simulink library "uavsimBlockset_UAV3D_visualizeBox"  (Simulink 8.6)
settings: Solver=ode45  StartTime=0.0  StopTime=10.0  RelTol=1e-3
libraries: aerolibtransform2 x1, uavsimBlockset_UAV3DInterface x1
settings Model: Creator=mstolle  LastModifiedBy=j.bolting

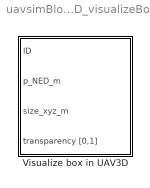
== system uavsimBlockset_UAV3D_visualizeBox ==
  Visualize box in UAV3D : Subsystem  TreatAsAtomicUnit=on  SystemSampleTime=1/10

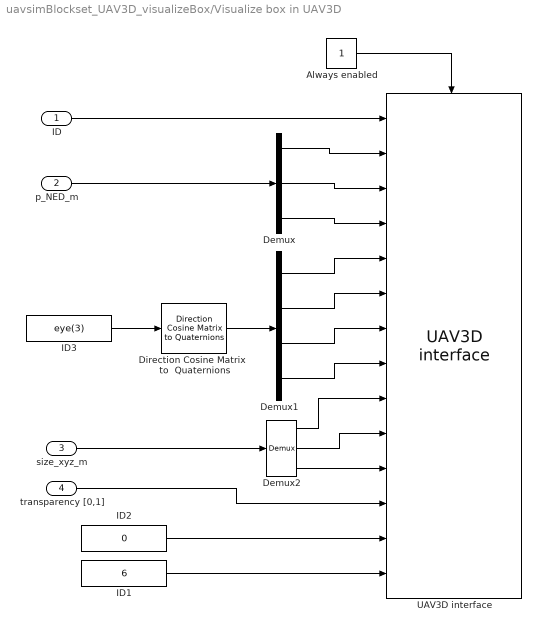
== system uavsimBlockset_UAV3D_visualizeBox/Visualize box in UAV3D ==
  ID : Inport
  p_NED_m : Inport  Port=2
  size_xyz_m : Inport  Port=3
  transparency [0,1] : Inport  Port=4
  Always enabled : Constant
  Demux : Demux  Outputs=3
  Demux1 : Demux
  Demux2 : Demux  Outputs=3
  Direction Cosine Matrix   to  Quaternions : aerolibtransform2/Direction Cosine Matrix  to Quaternions
  ID1 : Constant  Value=6
  ID2 : Constant  Value=0
  ID3 : Constant  Value=eye(3)
  UAV3D interface : uavsimBlockset_UAV3DInterface/UAV3D interface  ip='localhost'  udpport=4445
  wires:
  Always enabled/1 -> UAV3D interface/Enable
  transparency [0,1]/1 -> UAV3D interface/12
  Demux1/1 -> UAV3D interface/5
  Demux/2 -> UAV3D interface/3
  Demux/1 -> UAV3D interface/2
  Demux/3 -> UAV3D interface/4
  Demux1/2 -> UAV3D interface/6
  Demux1/3 -> UAV3D interface/7
  Demux1/4 -> UAV3D interface/8
  ID1/1 -> UAV3D interface/14
  ID/1 -> UAV3D interface/1
  Direction Cosine Matrix   to  Quaternions/1 -> Demux1/1
  p_NED_m/1 -> Demux/1
  ID2/1 -> UAV3D interface/13
  ID3/1 -> Direction Cosine Matrix   to  Quaternions/1
  Demux2/1 -> UAV3D interface/9
  Demux2/2 -> UAV3D interface/10
  size_xyz_m/1 -> Demux2/1
  Demux2/3 -> UAV3D interface/11
